simulink model "px4demo_LEDBuzzer"  (R2019b)
settings: Solver=FixedStepAuto  StartTime=0.0  StopTime=inf  RelTol=1e-3  EnableMultiTasking=on
undefined symbols (not defined in the file or in its folder): color, frequency, led_mask, mode, strength, tune_id, tune_override
libraries: px4uORBlib x4
settings Model: SimulationMode=external  ExtModeTrigDuration=10  Creator=The MathWorks, Inc.  LastModifiedBy=The MathWorks, Inc.
settings SolverCC: PositivePriorityOrder=on
settings OptimizationCC: EnhancedBackFolding=on  PassReuseOutputArgsAs=Individual arguments  ZeroExternalMemoryAtStartup=off  ZeroInternalMemoryAtStartup=off  MaxStackSize=64  OptimizeBlockOrder=speed  DifferentSizesBufferReuse=on  OptimizationCustomize=off  EfficientTunableParamExpr=on
settings DebuggingCC: ParameterTunabilityLossMsg=error
settings HardwareCC: ProdBitPerPointer=32  ProdBitPerSizeT=32  ProdBitPerPtrDiffT=32  ProdLargestAtomicInteger=Long  ProdLargestAtomicFloat=Double  ProdWordSize=32  ProdLongLongMode=on  ProdHWDeviceType=ARM Compatible->ARM Cortex
settings SFSimCC: MATLABDynamicMemAlloc=off
settings RTWCC: SystemTargetFile=ert.tlc  HardwareBoard=PX4 Pixhawk 1  TLCOptions="-aInlineSetEventsForThisBaseRateFcn=TLC_FALSE -aSuppressMultiTaskScheduler=TLC_FALSE  -aRateBasedStepFcn=0"  TemplateMakefile=ert_default_tmf  GenerateReport=on  Toolchain=GNU Tools for PX4 Autopilots  IncludeHyperlinkInReport=on  LaunchReport=on  TargetLang=C++  GenerateTraceInfo=on  GenerateTraceReport=on  GenerateTraceReportSl=on  GenerateTraceReportSf=on  GenerateTraceReportEml=on
settings CodeAppCC: ForceParamTrailComments=on  IgnoreCustomStorageClasses=off  OperatorAnnotations=on  SimulinkDataObjDesc=on  SFDataObjDesc=on  InsertBlockDesc=on

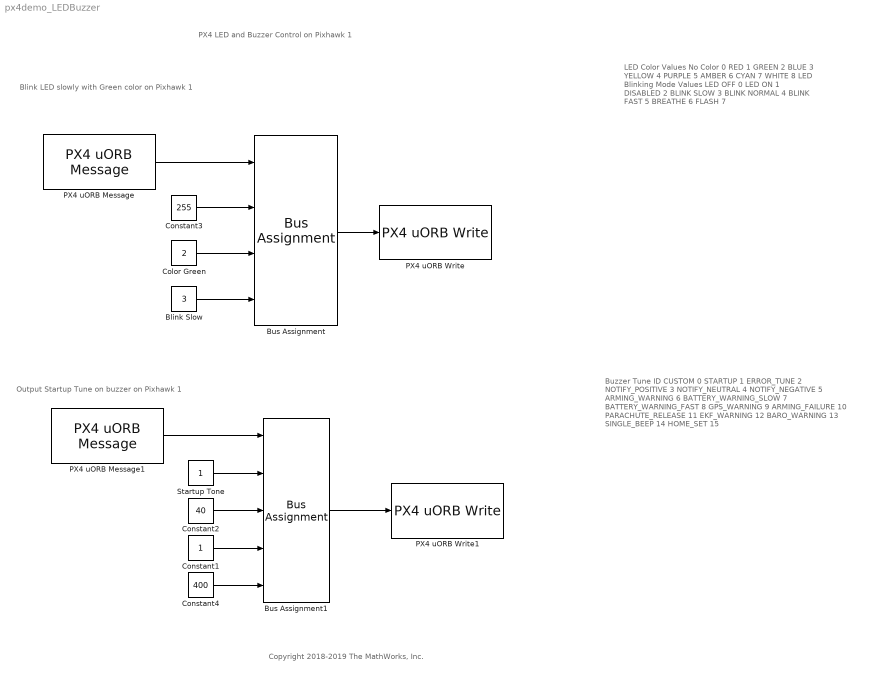
== system px4demo_LEDBuzzer ==
  note: LED Color Values
      |
      | No Color 0
      | RED 1
      | GREEN 2
      | BLUE 3
      | YELLOW 4
      | PURPLE 5
      | AMBER 6
      | CYAN 7
      | WHITE 8
      |
      | LED Blinking Mode Values
      | LED OFF 0
      | LED ON 1
      | DISABLED 2
      | BLINK SLOW 3
      | BLINK NORMAL 4
      | BLINK FAST 5
      | BREATHE 6
      | FLASH 7
  note: Output Startup Tune on buzzer on Pixhawk 1
  note: Copyright 2018-2019 The MathWorks, Inc.
  note: PX4 LED and Buzzer Control on Pixhawk 1
  note: Blink LED slowly with Green color on Pixhawk 1
  note: Buzzer Tune ID
      |
      | CUSTOM 0
      | STARTUP 1
      | ERROR_TUNE 2
      | NOTIFY_POSITIVE 3
      | NOTIFY_NEUTRAL 4
      | NOTIFY_NEGATIVE 5
      | ARMING_WARNING 6
      | BATTERY_WARNING_SLOW 7
      | BATTERY_WARNING_FAST 8
      | GPS_WARNING 9
      | ARMING_FAILURE 10
      | PARACHUTE_RELEASE 11
      | EKF_WARNING 12
      | BARO_WARNING 13
      | SINGLE_BEEP 14
      | HOME_SET 15
  Blink Slow : Constant  Value=3  OutDataTypeStr=Inherit: Inherit via back propagation  SampleTime=1
  Bus Assignment : BusAssignment  AssignedSignals=led_mask,color,mode
  Bus Assignment1 : BusAssignment  AssignedSignals=tune_id,strength,tune_override,frequency
  Color Green : Constant  Value=2  OutDataTypeStr=Inherit: Inherit via back propagation  SampleTime=1
  Constant1 : Constant  OutDataTypeStr=Inherit: Inherit via back propagation  SampleTime=1
  Constant2 : Constant  Value=40  OutDataTypeStr=Inherit: Inherit via back propagation  SampleTime=1
  Constant3 : Constant  Value=255  OutDataTypeStr=Inherit: Inherit via back propagation  SampleTime=1
  Constant4 : Constant  Value=400  OutDataTypeStr=Inherit: Inherit via back propagation  SampleTime=1
  PX4 uORB Message : px4uORBlib/PX4 uORB Message  uORBTopic=led_control  SampleTime=inf
      settings: SourceProductName=Embedded Coder Support Package for PX4 Autopilots  SourceProductBaseCode=PX4AUTOPILOTS
  PX4 uORB Message1 : px4uORBlib/PX4 uORB Message  uORBTopic=tune_control  SampleTime=inf
      settings: SourceProductName=Embedded Coder Support Package for PX4 Autopilots  SourceProductBaseCode=PX4AUTOPILOTS
  PX4 uORB Write : px4uORBlib/PX4 uORB Write  uORBTopic=led_control  MessageQueueLen=1
      settings: SourceProductName=Embedded Coder Support Package for PX4 Autopilots  SourceProductBaseCode=PX4AUTOPILOTS
  PX4 uORB Write1 : px4uORBlib/PX4 uORB Write  uORBTopic=tune_control  MessageQueueLen=1
      settings: SourceProductName=Embedded Coder Support Package for PX4 Autopilots  SourceProductBaseCode=PX4AUTOPILOTS
  Startup Tone : Constant  OutDataTypeStr=Inherit: Inherit via back propagation  SampleTime=1
  wires:
  Constant3/1 -> Bus Assignment/2
  PX4 uORB Message/1 -> Bus Assignment/1
  Blink Slow/1 -> Bus Assignment/4
  Color Green/1 -> Bus Assignment/3
  Bus Assignment/1 -> PX4 uORB Write/1
  PX4 uORB Message1/1 -> Bus Assignment1/1
  Bus Assignment1/1 -> PX4 uORB Write1/1
  Startup Tone/1 -> Bus Assignment1/2
  Constant2/1 -> Bus Assignment1/3
  Constant1/1 -> Bus Assignment1/4
  Constant4/1 -> Bus Assignment1/5
